simulink model "off_grid_voltage_filter"  (R2015b)
settings: Solver=VariableStepAuto  StartTime=0.0  StopTime=20  RelTol=1e-6
InitFcn:
  | ref=400;
  | v1=150;
  | v2=250;
libraries: powerlib x46, powerlib_meascontrol x7
settings Model: Creator=fujitsu  LastModifiedBy=fujitsu

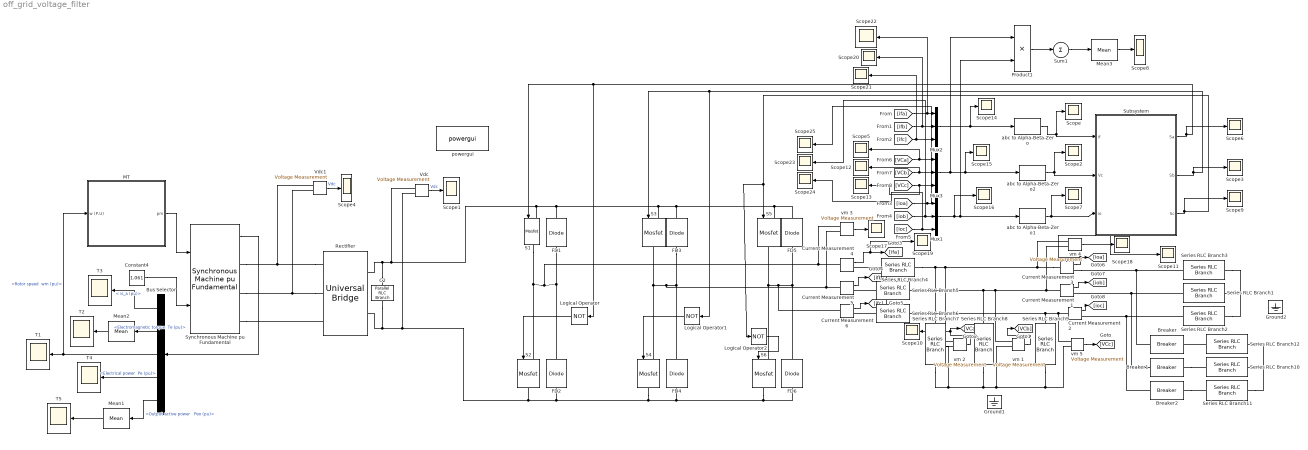
== system off_grid_voltage_filter ==
  Breaker : powerlib/Elements/Breaker  InitialState=0  SwitchingTimes=[15]  External=off  BreakerResistance=0.01  SnubberResistance=1e6  SnubberCapacitance=inf  Measurements=None  MoreParameters=on  NoBreakLoop=off
  Breaker1 : powerlib/Elements/Breaker  InitialState=0  SwitchingTimes=[15]  External=off  BreakerResistance=0.01  SnubberResistance=1e6  SnubberCapacitance=inf  Measurements=None  MoreParameters=on  NoBreakLoop=off
  Breaker2 : powerlib/Elements/Breaker  InitialState=0  SwitchingTimes=[15]  External=off  BreakerResistance=0.01  SnubberResistance=1e6  SnubberCapacitance=inf  Measurements=None  MoreParameters=on  NoBreakLoop=off
  Bus Selector : BusSelector  OutputSignals="Stator current. is_a (pu),Mechanical.Electromagnetic torque  Te (pu),Mechanical.Rotor speed  wm (pu),Mechanical.Electrical power  Pe (pu),Output active power   Peo (pu)"
  C2 : powerlib/Elements/Parallel RLC Branch  LConnTagsString=a  RConnTagsString=__new0  BranchType=C  Resistance=inf  Inductance=inf  SetiL0=off  InitialCurrent=0  Capacitance=5000e-06  Setx0=off  InitialVoltage=0  Measurements=None
  Constant4 : Constant  Value=1.061
  Current Measurement{1..6} (6 alike) : powerlib/Measurements/Current Measurement  PhasorSimulation=off  OutputType=Complex  PSBequivalent=0
  FD{1..6} (6 alike) : powerlib/Power Electronics/Diode  Ron=0.001  Lon=0  Vf=0.8  IC=0  UseSnubber=off  Rs=500  Cs=250e-9  Measurements=off
  Ground1 : powerlib/Elements/Ground  LConnTagsString=a
  Ground2 : powerlib/Elements/Ground  LConnTagsString=a
  Logical Operator : Logic  Operator=NOT  AllPortsSameDT=off  OutDataTypeStr=boolean
  Logical Operator1 : Logic  Operator=NOT  AllPortsSameDT=off  OutDataTypeStr=boolean
  Logical Operator2 : Logic  Operator=NOT  AllPortsSameDT=off  OutDataTypeStr=boolean
  MT : Subsystem
  Mean1 : powerlib_meascontrol/Measurements/Mean  Freq=50  Vinit=0  Ts=50e-6
  Mean2 : powerlib_meascontrol/Measurements/Mean  Freq=50  Vinit=0  Ts=50e-6
  Mean3 : powerlib_meascontrol/Measurements/Mean  Freq=50  Vinit=0  Ts=50e-6
  Mux1 : Mux  Inputs=3
  Mux2 : Mux  Inputs=3
  Mux3 : Mux  Inputs=3
  Product1 : Product  SaturateOnIntegerOverflow=on  InputSameDT=on  OutDataTypeStr=Inherit: Same as first input
  Rectifier : powerlib/Power Electronics/Universal Bridge  Arms=3  SnubberResistance=50  SnubberCapacitance=0.1e-6  Device=Diodes  Ron=1e-3  Lon=0  ForwardVoltages="[  0.8  0.8  ]"  ForwardVoltage=.7  GTOparameters=[ 10e-6 , 20e-6 ]  IGBTparameters=[ 1e-6 , 2e-6 ]  Measurements=Device currents  Measurements_2=None  converterType=Rectifier
  S{1..6} (6 alike) : powerlib/Power Electronics/Mosfet  Ron=0.1  Lon=0  Rd=0.01  Vfd=0  IC=0  Rs=1e5  Cs=inf  Measurements=off
  Scope{,1..25} (26 alike) : Scope
  Series RLC Branch{1..3,10..12} (6 alike) : powerlib/Elements/Series RLC Branch  LConnTagsString=__new0  RConnTagsString=__new0  BranchType=R  Resistance=50  Inductance=10e-3  SetiL0=off  InitialCurrent=0  Capacitance=1e-6  Setx0=off  InitialVoltage=0  Measurements=None
  Series RLC Branch4 : powerlib/Elements/Series RLC Branch  LConnTagsString=__new0  RConnTagsString=__new0  BranchType=L  Resistance=5  Inductance=3e-3  SetiL0=off  InitialCurrent=0  Capacitance=1e-6  Setx0=off  InitialVoltage=0  Measurements=None
  Series RLC Branch5 : powerlib/Elements/Series RLC Branch  LConnTagsString=__new0  RConnTagsString=__new0  BranchType=L  Resistance=5  Inductance=3e-3  SetiL0=off  InitialCurrent=0  Capacitance=1e-6  Setx0=off  InitialVoltage=0  Measurements=None
  Series RLC Branch6 : powerlib/Elements/Series RLC Branch  LConnTagsString=__new0  RConnTagsString=__new0  BranchType=L  Resistance=5  Inductance=3e-3  SetiL0=off  InitialCurrent=0  Capacitance=1e-6  Setx0=off  InitialVoltage=0  Measurements=None
  Series RLC Branch7 : powerlib/Elements/Series RLC Branch  LConnTagsString=__new0  RConnTagsString=__new0  BranchType=C  Resistance=5  Inductance=10e-3  SetiL0=off  InitialCurrent=0  Capacitance=50e-6  Setx0=off  InitialVoltage=0  Measurements=None
  Series RLC Branch8 : powerlib/Elements/Series RLC Branch  LConnTagsString=__new0  RConnTagsString=__new0  BranchType=C  Resistance=5  Inductance=10e-3  SetiL0=off  InitialCurrent=0  Capacitance=50e-6  Setx0=off  InitialVoltage=0  Measurements=None
  Series RLC Branch9 : powerlib/Elements/Series RLC Branch  LConnTagsString=__new0  RConnTagsString=__new0  BranchType=C  Resistance=5  Inductance=10e-3  SetiL0=off  InitialCurrent=0  Capacitance=50e-6  Setx0=off  InitialVoltage=0  Measurements=None
  Subsystem : Subsystem
  Sum1 : Sum  Inputs=1  SaturateOnIntegerOverflow=on  InputSameDT=on  OutDataTypeStr=Inherit: Same as first input
  Synchronous Machine pu Fundamental : powerlib/Machines/Synchronous Machine pu Fundamental  PresetModel=No  MechanicalLoad=Mechanical power Pm  ShowDetailedParameters=on  RotorType=Salient-pole  Units=per unit fundamental parameters  MeasurementBus=off  NominalParameters="[ 65e3  600 1600]"  Stator="[ 0.2503  0.114  0.6875  0.6875 ]"  Field="[ 1  10e15/(100*pi)]"  Dampers2=[0.0652, 0.5134, 0.0287, 0.2553, 7.765e-3, 0.9167 ]  Dampers1="[ 1.17E-02  0.182  1.97E-02  0.384 ]"  Mechanical=[ 6 0 2]  PolePairs=20  InitialConditions="[ 0  0  0  0  0  0  0  0  1 ]"  SetSaturation=off  Saturation=[0.6404,0.7127,0.8441,0.9214,0.9956,1.082,1.19,1.316,1.457;0.7,0.7698,0.8872,0.9466,0.9969,1.046,1.1,1.151,1.201]  LoadFlowParameters=[1,0,0,0,0]  TsPowergui=0  TsBlock=-1  IterativeModel=Trapezoidal non iterative  BusType=swing  Pref=0  Qref=0  Qmin=-inf  Qmax=inf  PLF=0  QLF=0
  T{1..5} (5 alike) : Scope
  Vdc : powerlib/Measurements/Voltage Measurement  Tag=PoWeRsYsTeMmEaSuReMeNt  PhasorSimulation=off  OutputType=Magnitude  PSBequivalent=0
  Vdc1 : powerlib/Measurements/Voltage Measurement  Tag=PoWeRsYsTeMmEaSuReMeNt  PhasorSimulation=off  OutputType=Magnitude  PSBequivalent=0
  abc to Alpha-Beta-Zero : powerlib_meascontrol/Transformations/abc to Alpha-Beta-Zero
  abc to Alpha-Beta-Zero1 : powerlib_meascontrol/Transformations/abc to Alpha-Beta-Zero
  abc to Alpha-Beta-Zero2 : powerlib_meascontrol/Transformations/abc to Alpha-Beta-Zero
  powergui : powerlib/powergui  SimulationMode=Discrete  SolverType=Tustin  SampleTime=1e-6  frequency=60  SPID=off  DisableSnubberDevices=off  DisableRonSwitches=off  DisableVfSwitches=off  SwTol=0  DisplayEquations=off  Interpol=off  ExternalGateDelay=off  methode=off  Ts=0  FunctionMessages=off  echomessages=off  HookPort=off  EnableUseOfTLC=off  x0status=blocks  frequencyindice=0  Pbase=100e6  ErrMax=0.0001  Iterations=50  UnitsV=kV  UnitsW=MW  buscounter=0  RestoreLinks=warning  ResistiveCurrentMeasurement=off  Frange=[0:2:500]  Ylog=off  Xlog=on  ShowGrid=off  save=off  variable=ZData  structure=vca  ZoomFFT=off  StartTime=0.04  cycles=3  DisplayStyle=1  fundamental=50  FreqAxis=on  MaxFrequency=10000  frequencyindicesteady=1  RmsSteady=1  display=off
  vm {1..5} (5 alike) : powerlib/Measurements/Voltage Measurement  PhasorSimulation=off  OutputType=Complex  PSBequivalent=0
  wires:
  Vdc/1 -> Scope1/1  "Vdc"
  MT/1(pm) -> Synchronous Machine pu Fundamental/1
  Synchronous Machine pu Fundamental/1 -> Bus Selector/1
  Bus Selector/1 -> T3/1  "< is_a (pu)>"
  Bus Selector/3 -> MT/1(w (P.U)), T1/1  "<Rotor speed  wm (pu)>"
  Constant4/1 -> Synchronous Machine pu Fundamental/2
  Vdc1/1 -> Scope4/1  "Vdc"
  Bus Selector/4 -> T4/1  "<Electrical power  Pe (pu)>"
  Bus Selector/5 -> Mean1/1  "<Output active power   Peo (pu)>"
  Mean1/1 -> T5/1
  Logical Operator/1 -> S2/1
  Logical Operator1/1 -> S4/1
  Logical Operator2/1 -> S6/1
  vm 5/1 -> [VCc]
  vm 1/1 -> [VCb]
  vm 2/1 -> [VCa], Scope10/1
  Current Measurement4/1 -> Scope19/1, [ifa]
  Current Measurement5/1 -> [ifb]
  Current Measurement6/1 -> [ifc]
  Current Measurement3/1 -> [ioa], Scope11/1
  Current Measurement1/1 -> [iob]
  Current Measurement2/1 -> [ioc]
  Mux2/1 -> Scope14/1, abc to Alpha-Beta-Zero/1
  [ifa] -> Scope22/1, Mux2/1
  [ifb] -> Mux2/2, Scope20/1
  [ifc] -> Mux2/3, Scope21/1
  Mux1/1 -> Scope16/1, Product1/2, abc to Alpha-Beta-Zero1/1
  [ioa] -> Scope25/1, Mux1/1
  [iob] -> Scope23/1, Mux1/2
  [ioc] -> Scope24/1, Mux1/3
  Mux3/1 -> Product1/1, Scope15/1, abc to Alpha-Beta-Zero2/1
  [VCa] -> Scope5/1, Mux3/1
  [VCb] -> Scope12/1, Mux3/2
  [VCc] -> Scope13/1, Mux3/3
  abc to Alpha-Beta-Zero/1 -> Scope/1, Subsystem/1(if)
  abc to Alpha-Beta-Zero2/1 -> Scope2/1, Subsystem/2(Vc)
  abc to Alpha-Beta-Zero1/1 -> Scope7/1, Subsystem/3(io)
  Subsystem/1(Sa) -> Scope6/1, Logical Operator/1, S1/1
  Subsystem/2(Sb) -> Scope3/1, Logical Operator1/1, S3/1
  Subsystem/3(Sc) -> Scope9/1, Logical Operator2/1, S5/1
  vm 3/1 -> Scope17/1
  vm 4/1 -> Scope18/1
  Mean3/1 -> Scope8/1
  Sum1/1 -> Mean3/1
  Product1/1 -> Sum1/1
  Mean2/1 -> T2/1
  Bus Selector/2 -> Mean2/1  "<Electromagnetic torque  Te (pu)>"
  connections:
  Rectifier/LConn1 -- Synchronous Machine pu Fundamental/RConn1 -- Vdc1/LConn1
  Rectifier/LConn2 -- Synchronous Machine pu Fundamental/RConn2 -- Vdc1/LConn2
  Synchronous Machine pu Fundamental/RConn3 -- Rectifier/LConn3
  C2/LConn1 -- Rectifier/RConn1 -- FD1/RConn1 -- S3/LConn1 -- FD3/RConn1 -- FD5/RConn1 -- S5/LConn1 -- S1/LConn1 -- Vdc/LConn1
  Rectifier/RConn2 -- C2/RConn1 -- S2/RConn1 -- FD2/LConn1 -- S4/RConn1 -- S6/RConn1 -- FD6/LConn1 -- FD4/LConn1 -- Vdc/LConn2
  S1/RConn1 -- S2/LConn1 -- vm 3/LConn1 -- Current Measurement4/LConn1 -- FD1/LConn1 -- FD2/RConn1
  S3/RConn1 -- S4/LConn1 -- vm 3/LConn2 -- Current Measurement5/LConn1 -- FD3/LConn1 -- FD4/RConn1
  FD6/RConn1 -- FD5/LConn1 -- Current Measurement6/LConn1 -- S5/RConn1 -- S6/LConn1
  Series RLC Branch3/RConn1 -- Series RLC Branch2/RConn1 -- Series RLC Branch1/RConn1
  Current Measurement3/LConn1 -- vm 4/LConn1 -- Series RLC Branch7/LConn1 -- Series RLC Branch4/RConn1 -- vm 2/LConn1
  vm 1/LConn1 -- Series RLC Branch5/RConn1 -- Series RLC Branch8/LConn1 -- vm 4/LConn2 -- Current Measurement1/LConn1
  Current Measurement2/LConn1 -- Series RLC Branch6/RConn1 -- Series RLC Branch9/LConn1 -- vm 5/LConn1
  vm 1/LConn2 -- Series RLC Branch8/RConn1 -- Series RLC Branch7/RConn1 -- vm 2/LConn2 -- Series RLC Branch9/RConn1 -- vm 5/LConn2
  Current Measurement3/RConn1 -- Breaker/LConn1 -- Series RLC Branch3/LConn1
  Series RLC Branch6/LConn1 -- Current Measurement6/RConn1
  Series RLC Branch1/LConn1 -- Breaker1/LConn1 -- Current Measurement1/RConn1
  Series RLC Branch5/LConn1 -- Current Measurement5/RConn1
  Series RLC Branch2/LConn1 -- Breaker2/LConn1 -- Current Measurement2/RConn1
  Series RLC Branch4/LConn1 -- Current Measurement4/RConn1
  Series RLC Branch12/RConn1 -- Series RLC Branch11/RConn1 -- Series RLC Branch10/RConn1
  Series RLC Branch12/LConn1 -- Breaker/RConn1
  Breaker1/RConn1 -- Series RLC Branch10/LConn1
  Breaker2/RConn1 -- Series RLC Branch11/LConn1

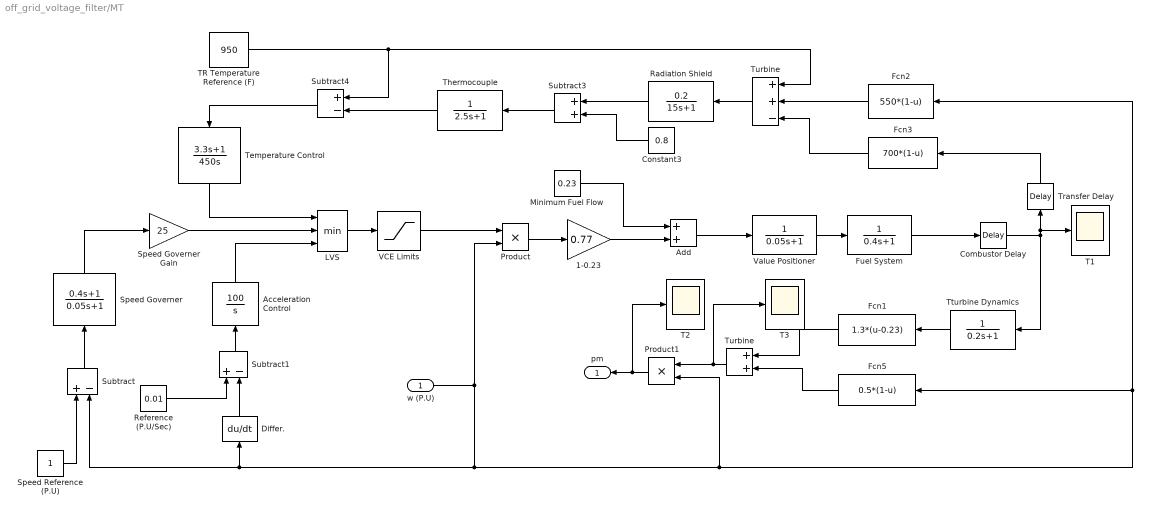
== system off_grid_voltage_filter/MT ==
  w (P.U) : Inport
  1-0.23 : Gain  Gain=0.77
  Acceleration Control : TransferFcn  Numerator=[0 100]  Denominator=[1 0]
  Add : Sum
  Combustor Delay : TransportDelay  DelayTime=0.01
  Constant3 : Constant  Value=0.8
  Differ. : Derivative
  Fcn1 : Fcn  Expr=1.3*(u-0.23)
  Fcn2 : Fcn  Expr=550*(1-u)
  Fcn3 : Fcn  Expr=700*(1-u)
  Fcn5 : Fcn  Expr=0.5*(1-u)
  Fuel System : TransferFcn  Denominator=[0.4 1]
  LVS : MinMax  Inputs=3
  Minimum Fuel Flow : Constant  Value=0.23
  Product : Product  RndMeth=Zero
  Product1 : Product  RndMeth=Zero
  Radiation Shield : TransferFcn  Numerator=[0.2]  Denominator=[15 1]
  Reference (P.U/Sec) : Constant  Value=0.01
  Speed Governer : TransferFcn  Numerator=[0.4 1]  Denominator=[0.05 1]
  Speed Governer Gain : Gain  Gain=25
  Speed Reference (P.U) : Constant
  Subtract : Sum  Inputs=+-
  Subtract1 : Sum  Inputs=+-
  Subtract3 : Sum
  Subtract4 : Sum  Inputs=+-
  T1 : Scope
  T2 : Scope
  T3 : Scope
  TR Temperature Reference (F) : Constant  Value=950
  Temperature Control : TransferFcn  Numerator=[3.3 1]  Denominator=[450 0]
  Thermocouple : TransferFcn  Denominator=[2.5 1]
  Transfer Delay : TransportDelay  DelayTime=0.04
  Tturbine Dynamics : TransferFcn  Denominator=[0.2 1]
  Turbine : Sum  Inputs=++-
  "Turbine " : Sum
  VCE Limits : Saturate  UpperLimit=1.5  LowerLimit=-0.1
  Value Positioner : TransferFcn  Denominator=[0.05 1]
  pm : Outport
  wires:
  Speed Reference (P.U)/1 -> Subtract/1
  Subtract/1 -> Speed Governer/1
  VCE Limits/1 -> Product/1
  Product/1 -> 1-0.23/1
  1-0.23/1 -> Add/2
  Minimum Fuel Flow/1 -> Add/1
  Add/1 -> Value Positioner/1
  Value Positioner/1 -> Fuel System/1
  Fuel System/1 -> Combustor Delay/1
  Combustor Delay/1 -> T1/1, Transfer Delay/1, Tturbine Dynamics/1
  Speed Governer Gain/1 -> LVS/2
  Differ./1 -> Subtract1/2
  Reference (P.U/Sec)/1 -> Subtract1/1
  Subtract1/1 -> Acceleration Control/1
  Acceleration Control/1 -> LVS/3
  LVS/1 -> VCE Limits/1
  Transfer Delay/1 -> Fcn3/1
  Fcn3/1 -> Turbine/3
  Fcn2/1 -> Turbine/2
  Radiation Shield/1 -> Subtract3/1
  Constant3/1 -> Subtract3/2
  Turbine/1 -> Radiation Shield/1
  Subtract3/1 -> Thermocouple/1
  Thermocouple/1 -> Subtract4/2
  TR Temperature Reference (F)/1 -> Turbine/1, Subtract4/1
  Subtract4/1 -> Temperature Control/1
  Temperature Control/1 -> LVS/1
  Speed Governer/1 -> Speed Governer Gain/1
  w (P.U)/1 -> Product/2, Subtract/2, Differ./1, Product1/2, Fcn5/1, Fcn2/1
  Tturbine Dynamics/1 -> Fcn1/1
  Fcn1/1 -> "Turbine "/1
  Fcn5/1 -> "Turbine "/2
  "Turbine "/1 -> Product1/1, T3/1
  Product1/1 -> T2/1, pm/1

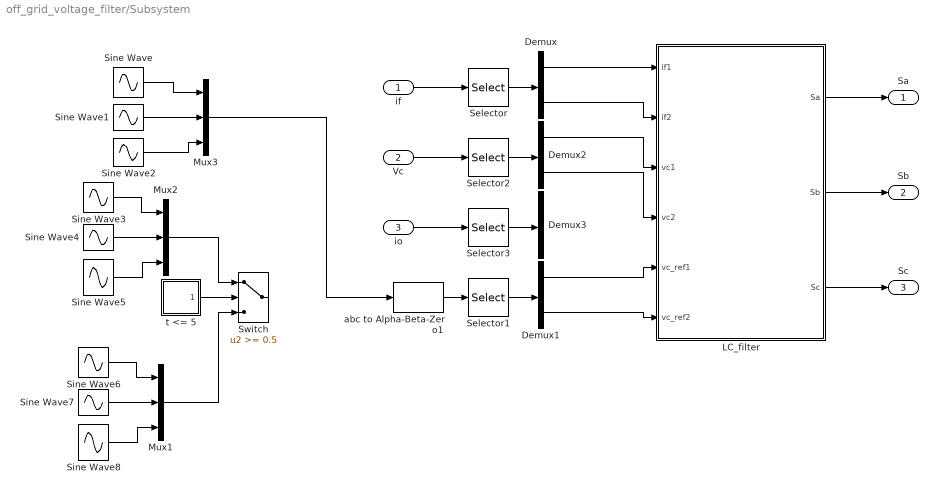
== system off_grid_voltage_filter/Subsystem ==
  if : Inport
  Vc : Inport  Port=2
  io : Inport  Port=3
  Demux{,1..3} (4 alike) : Demux  Outputs=2
  LC_filter : MATLAB Function  TreatAsAtomicUnit=on
  Mux1 : Mux  Inputs=3
  Mux2 : Mux  Inputs=3
  Mux3 : Mux  Inputs=3
  Selector{,1..3} (4 alike) : Selector  InputPortWidth=3  IndexOptions=Index vector (dialog)  Indices=[1 2]  OutputSizes=1
  Sine Wave : Sin  Amplitude=ref  Frequency=2*pi*50  SampleTime=0
  Sine Wave1 : Sin  Amplitude=ref  Frequency=100*pi  Phase=-2*pi/3  SampleTime=0
  Sine Wave2 : Sin  Amplitude=ref  Frequency=100*pi  Phase=+2*pi/3  SampleTime=0
  Sine Wave3 : Sin  Amplitude=v1  Frequency=2*pi*50  SampleTime=0
  Sine Wave4 : Sin  Amplitude=v1  Frequency=100*pi  Phase=-2*pi/3  SampleTime=0
  Sine Wave5 : Sin  Amplitude=v1  Frequency=100*pi  Phase=2*pi/3  SampleTime=0
  Sine Wave6 : Sin  Amplitude=v2  Frequency=2*pi*50  SampleTime=0
  Sine Wave7 : Sin  Amplitude=v2  Frequency=100*pi  Phase=-2*pi/3  SampleTime=0
  Sine Wave8 : Sin  Amplitude=v2  Frequency=100*pi  Phase=2*pi/3  SampleTime=0
  Switch : Switch  Threshold=0.5  SaturateOnIntegerOverflow=on  InputSameDT=on
  abc to Alpha-Beta-Zero1 : powerlib_meascontrol/Transformations/abc to Alpha-Beta-Zero
  t <= 5 : Subsystem
  Sa : Outport
  Sb : Outport  Port=2
  Sc : Outport  Port=3
  wires:
  Selector/1 -> Demux/1
  abc to Alpha-Beta-Zero1/1 -> Selector1/1
  Sine Wave/1 -> Mux3/1
  Sine Wave1/1 -> Mux3/2
  Sine Wave2/1 -> Mux3/3
  if/1 -> Selector/1
  LC_filter/1(Sa) -> Sa/1
  LC_filter/2(Sb) -> Sb/1
  LC_filter/3(Sc) -> Sc/1
  Demux/1 -> LC_filter/1(if1)
  Demux/2 -> LC_filter/2(if2)
  Selector2/1 -> Demux2/1
  Selector3/1 -> Demux3/1
  Vc/1 -> Selector2/1
  Demux2/1 -> LC_filter/3(vc1)
  Demux2/2 -> LC_filter/4(vc2)
  io/1 -> Selector3/1
  Demux1/1 -> LC_filter/5(vc_ref1)
  Demux1/2 -> LC_filter/6(vc_ref2)
  Selector1/1 -> Demux1/1
  t <= 5/1(t <= 1) -> Switch/2
  Sine Wave3/1 -> Mux2/1
  Sine Wave4/1 -> Mux2/2
  Sine Wave5/1 -> Mux2/3
  Sine Wave6/1 -> Mux1/1
  Sine Wave7/1 -> Mux1/2
  Sine Wave8/1 -> Mux1/3
  Mux2/1 -> Switch/1
  Mux1/1 -> Switch/3
  Mux3/1 -> abc to Alpha-Beta-Zero1/1

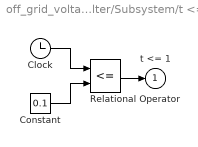
== system off_grid_voltage_filter/Subsystem/t <= 5 ==
  Clock : Clock
  Constant : Constant  Value=0.1
  Relational Operator : RelationalOperator  Operator=<=  InputSameDT=on
  t <= 1 : Outport  InitialOutput=0
  wires:
  Constant/1 -> Relational Operator/2
  Clock/1 -> Relational Operator/1
  Relational Operator/1 -> t <= 1/1

== matlab function off_grid_voltage_filter/Subsystem/LC_filter ==
  data: if1 input; Sa output; if2 input; vc1 input; vc2 input; Sb output; Sc output; vc_ref1 input; vc_ref2 input
function [Sa,Sb,Sc]=LC(if1,if2,vc1,vc2,vc_ref1,vc_ref2)
T=25e-6;
c=50e-6;
Aq=[0.9979  -0.008328;0.4997     0.9979];
Bq=[0.008328  0.002083;0.002083   -0.4997];
Vdc=700;
v0=0;
v1=2/3*Vdc;
v2=1/3*Vdc+1j*sqrt(3)/3*Vdc;
v3=-1/3*Vdc+1j*sqrt(3)/3*Vdc;
v4=-2/3*Vdc;
v5=-1/3*Vdc-1j*sqrt(3)/3*Vdc;
v6=1/3*Vdc-1j*sqrt(3)/3*Vdc;
v7=0;
v=[v0 v1 v2 v3 v4 v5 v6 v7]; %standars vector
states=[0 0 0;1 0 0;1 1 0;0 1 0;0 1 1;0 0 1;1 0 1;1 1 1]; %based on SVM standard vectors
persistent vc_old if_old io_old 
if isempty(vc_old), vc_old=0+1j*0; end
if isempty(if_old), if_old=0+1j*0; end
g=zeros(1,8); 
iff=if1+1j*if2;
vc=vc1+1j*vc2;
vc_ref=vc_ref1+1j*vc_ref2;
io_old=if_old-(c/T)*(vc-vc_old);
if_old=iff;
vc_old=vc;
io=io_old;
for i=1:8
v_o1=v(i); 
vcc=Aq(2,1)*iff+Aq(2,2)*vc+Bq(2,1)*v_o1+Bq(2,2)*io; 
g(i)=abs(real(vc_ref-vcc))+abs(imag(vc_ref-vcc)); 
end
[yy,x_opt]=min(g);%yy shows least value and x_opt shows colimn that is related to yy values.
Sa=states(x_opt,1);
Sb=states(x_opt,2);
Sc=states(x_opt,3);
